simulink model "Modulations-Simulink"  (R2020a)
settings: Solver=VariableStepAuto  StartTime=0.0  StopTime=10.0  RelTol=1e-3
libraries: dspsigops x1, powerlib_meascontrol x1
settings Model: Creator=Mert Beser  LastModifiedBy=Mert Beser

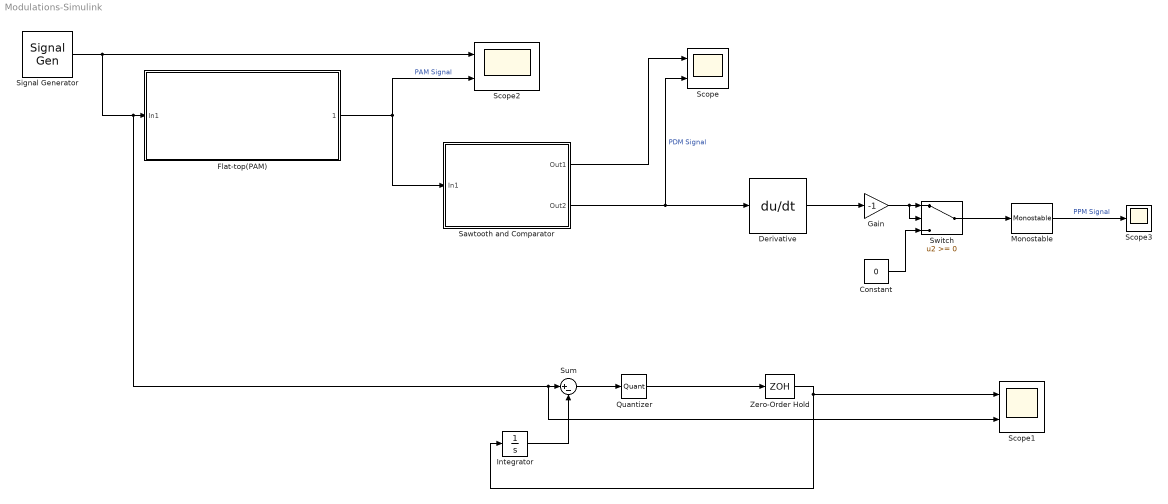
== system Modulations-Simulink ==
  Constant : Constant  Value=0
  Derivative : Derivative
  "Flat-top(PAM) " : Subsystem
  Gain : Gain  Gain=-1
  Integrator : Integrator
  Monostable : powerlib_meascontrol/Logic/Monostable  EdgeDetect=Rising  PulseDuration=0.2  ic=0  Ts=0
      settings: SourceProductBaseCode=PS
  Quantizer : Quantizer
  Sawtooth and Comparator : Subsystem
  Scope : Scope  NumInputPorts=2
  Scope1 : Scope  NumInputPorts=2
  Scope2 : Scope  NumInputPorts=2
  Scope3 : Scope
  Signal Generator : SignalGenerator  Frequency=1/4
  Sum : Sum  Inputs=|+-
  Switch : Switch
  Zero-Order Hold : ZeroOrderHold  SampleTime=-1
  wires:
  Signal Generator/1 -> Scope2/1, Scope1/2, Sum/1, "Flat-top(PAM) "/1(In1)
  "Flat-top(PAM) "/1(" ") -> Sawtooth and Comparator/1(In1), Scope2/2  "PAM Signal"
  Sawtooth and Comparator/1(Out1) -> Scope/1
  Sawtooth and Comparator/2(Out2) -> Derivative/1, Scope/2  "PDM Signal"
  Constant/1 -> Switch/3
  Gain/1 -> Switch/2, Switch/1
  Derivative/1 -> Gain/1
  Switch/1 -> Monostable/1
  Monostable/1 -> Scope3/1  "PPM Signal"
  Quantizer/1 -> Zero-Order Hold/1
  Zero-Order Hold/1 -> Scope1/1, Integrator/1
  Sum/1 -> Quantizer/1
  Integrator/1 -> Sum/2

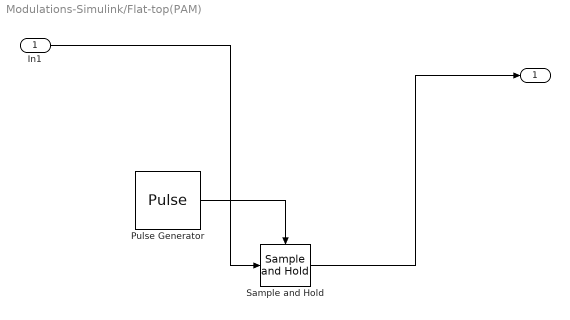
== system Modulations-Simulink/Flat-top(PAM)  ==
  In1 : Inport
  Pulse Generator : DiscretePulseGenerator  PulseType=Time based  Period=0.4  PulseWidth=50
  Sample and Hold : dspsigops/Sample and Hold  trig=Rising edge  initCond=0  latchinput=off
  " " : Outport
  wires:
  In1/1 -> Sample and Hold/1
  Pulse Generator/1 -> Sample and Hold/Trigger
  Sample and Hold/1 -> " "/1

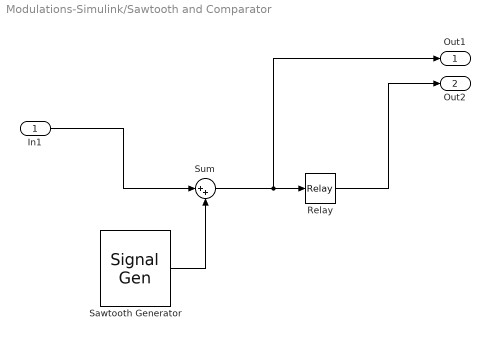
== system Modulations-Simulink/Sawtooth and Comparator ==
  In1 : Inport
  Relay : Relay
  Sawtooth Generator : SignalGenerator  WaveForm=sawtooth  Amplitude=1.5  Frequency=2
  Sum : Sum  Inputs=|++
  Out1 : Outport
  Out2 : Outport  Port=2
  wires:
  Sum/1 -> Out1/1, Relay/1
  Sawtooth Generator/1 -> Sum/2
  In1/1 -> Sum/1
  Relay/1 -> Out2/1
